simulink model "summator"  (R2023b)
settings: Solver=VariableStepAuto  StartTime=0.0  StopTime=10.0  RelTol=1e-3
settings Model: Creator=1234  LastModifiedBy=1234

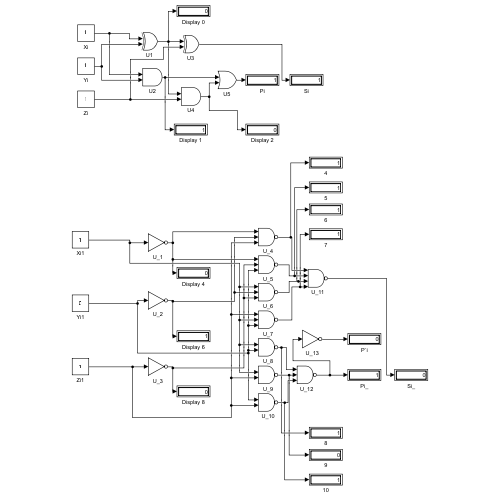
[thumbnail: Simulink's stored preview of the top-level diagram]
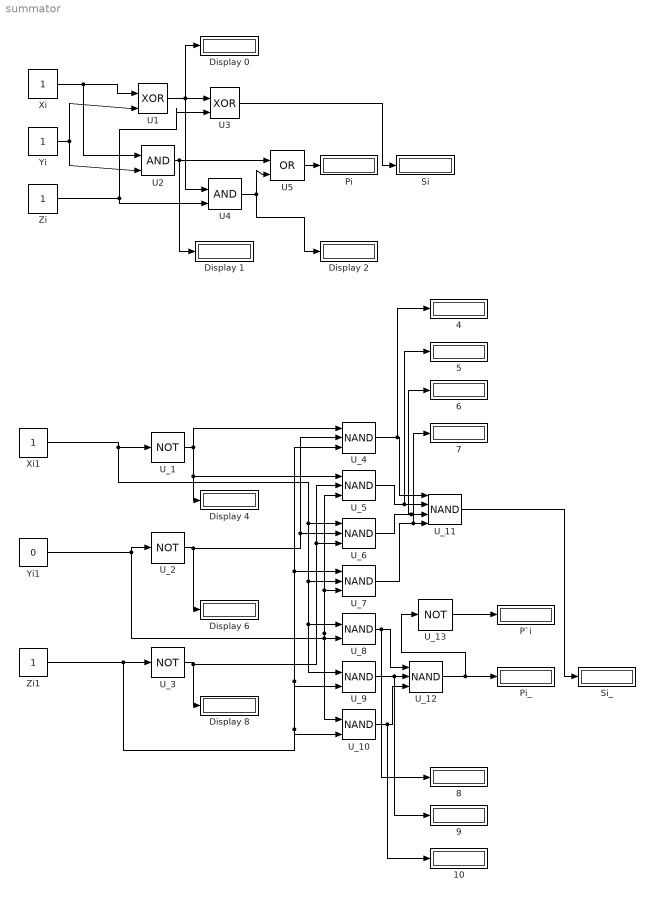
== system summator ==
  {4..10} (7 alike) : Display
  Display {0..2,4,6,8} (6 alike) : Display
  P`i : Display
  Pi : Display
  Pi_ : Display
  Si : Display
  Si_ : Display
  U1 : Logic  Operator=XOR  IconShape=distinctive  AllPortsSameDT=off  OutDataTypeStr=boolean
  U2 : Logic  IconShape=distinctive  AllPortsSameDT=off  OutDataTypeStr=boolean
  U3 : Logic  Operator=XOR  IconShape=distinctive  AllPortsSameDT=off  OutDataTypeStr=boolean
  U4 : Logic  IconShape=distinctive  AllPortsSameDT=off  OutDataTypeStr=boolean
  U5 : Logic  Operator=OR  IconShape=distinctive  AllPortsSameDT=off  OutDataTypeStr=boolean
  U_{1..3,13} (4 alike) : Logic  Operator=NOT  IconShape=distinctive  AllPortsSameDT=off  OutDataTypeStr=boolean
  U_10 : Logic  Operator=NAND  IconShape=distinctive  AllPortsSameDT=off  OutDataTypeStr=boolean
  U_11 : Logic  Operator=NAND  Inputs=4  IconShape=distinctive  AllPortsSameDT=off  OutDataTypeStr=boolean
  U_{4..7,12} (5 alike) : Logic  Operator=NAND  Inputs=3  IconShape=distinctive  AllPortsSameDT=off  OutDataTypeStr=boolean
  U_8 : Logic  Operator=NAND  IconShape=distinctive  AllPortsSameDT=off  OutDataTypeStr=boolean
  U_9 : Logic  Operator=NAND  IconShape=distinctive  AllPortsSameDT=off  OutDataTypeStr=boolean
  Xі : Constant
  Xі1 : Constant
  Yi : Constant
  Yi1 : Constant  Value=0
  Zi : Constant
  Zi1 : Constant
  wires:
  Xі/1 -> U1/1, U2/1
  Yi/1 -> U1/2, U2/2
  U1/1 -> Display 0/1, U4/1, U3/1
  Zi/1 -> U4/2, U3/2
  U3/1 -> Si/1
  U2/1 -> Display 1/1, U5/1
  U4/1 -> U5/2, Display 2/1
  U5/1 -> Pi/1
  Xі1/1 -> U_6/1, U_7/2, U_8/1, U_9/1, U_1/1
  Yi1/1 -> U_2/1, U_5/3, U_7/3, U_8/2, U_10/1
  Zi1/1 -> U_7/1, U_4/3, U_9/2, U_10/2, U_3/1
  U_3/1 -> U_6/3, U_5/2, Display 8/1
  U_2/1 -> U_6/2, U_4/2, Display 6/1
  U_1/1 -> U_4/1, U_5/1, Display 4/1
  U_4/1 -> 4/1, U_11/1
  U_5/1 -> 5/1, U_11/2
  U_6/1 -> 6/1, U_11/3
  U_7/1 -> 7/1, U_11/4
  U_9/1 -> 9/1, U_12/2
  U_8/1 -> 8/1, U_12/1
  U_11/1 -> Si_/1
  U_12/1 -> Pi_/1, U_13/1
  U_13/1 -> P`i/1
  U_10/1 -> 10/1, U_12/3
